simulink library "MyLib"  (R2016a)
settings: Solver=ode45  StartTime=0.0  StopTime=10.0  RelTol=1e-3
settings Model: Creator=NBGD  LastModifiedBy=NBGD
settings DataIOCC: LimitDataPoints=on
settings DebuggingCC: AllowSymbolicDim=off

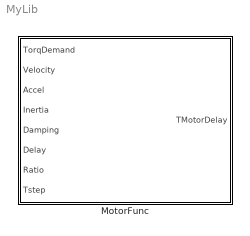
== system MyLib ==
  MotorFunc : Subsystem

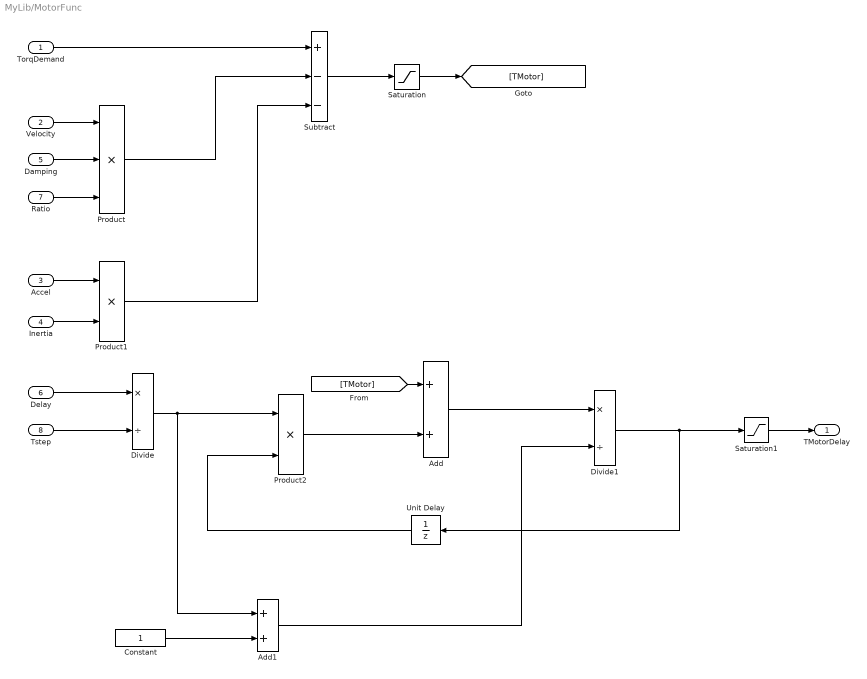
== system MyLib/MotorFunc ==
  TorqDemand : Inport
  Velocity : Inport  Port=2
  Accel : Inport  Port=3
  Inertia : Inport  Port=4
  Damping : Inport  Port=5
  Delay : Inport  Port=6
  Ratio : Inport  Port=7
  Tstep : Inport  Port=8
  Add : Sum
  Add1 : Sum
  Constant : Constant
  Divide : Product  Inputs=*/
  Divide1 : Product  Inputs=*/
  Product : Product  Inputs=3
  Product1 : Product
  Product2 : Product
  Saturation : Saturate  UpperLimit=300  LowerLimit=0
  Saturation1 : Saturate  UpperLimit=300  LowerLimit=0
  Subtract : Sum  Inputs=+--
  Unit Delay : UnitDelay  SampleTime=-1
  TMotorDelay : Outport
  wires:
  Velocity/1 -> Product/1
  Damping/1 -> Product/2
  Ratio/1 -> Product/3
  Accel/1 -> Product1/1
  Inertia/1 -> Product1/2
  TorqDemand/1 -> Subtract/1
  Product/1 -> Subtract/2
  Product1/1 -> Subtract/3
  Subtract/1 -> Saturation/1
  Delay/1 -> Divide/1
  Tstep/1 -> Divide/2
  Divide/1 -> Add1/1, Product2/1
  Unit Delay/1 -> Product2/2
  Product2/1 -> Add/2
  Add/1 -> Divide1/1
  [TMotor] -> Add/1
  Constant/1 -> Add1/2
  Add1/1 -> Divide1/2
  Divide1/1 -> Unit Delay/1, Saturation1/1
  Saturation/1 -> [TMotor]
  Saturation1/1 -> TMotorDelay/1
